simulink model "aero_gen"  (R2021b)
settings: Solver=ode45  StartTime=0.0  StopTime=inf  FixedStep=0.005  RelTol=1e-3
model workspace (MATLAB code in the model file + MAT data in the model file):
  | k = 110
values from neighbouring files (symbols this model uses):
  pitch_c = deg2rad(8)    [run_sim.m]    (also in run_sim_config.m = flight_config.aircraft_params.pitch_control_input; run_static_trim.m = deg2rad(-10))
  roll_c_1 = deg2rad(0)    [run_sim.m]    (also in run_sim_config.m = flight_config.aircraft_params.roll_control_input_1; run_static_trim.m = deg2rad(12.6))
  viz_on = 1    [run_sim.m]    (also in run_sim_config.m = flight_config.sys_params.viz_on; run_static_trim.m)
  yaw_moment_1 = 0.00    (= 0)    [run_sim.m]    (also in run_sim_config.m = flight_config.aircraft_params.yaw_moment_coeff_1; run_static_trim.m)
undefined symbols (not defined in the file or in its folder): state1
libraries: block_library x7, vrlib x1
settings Model: SnapshotBufferSize=1000  Creator=austm  LastModifiedBy=austm
settings SolverCC: ZeroCrossAlgorithm=Adaptive  AutoInsertRateTranBlk=on  InsertRTBMode=Never (minimum delay)  DecoupledContinuousIntegration=on  MinimalZcImpactIntegration=on
settings DataIOCC: ExternalInput=[0, u_trim']  InitialState=[x_trim']  LoadExternalInput=on  SaveFormat=Array  SaveOutput=off  ReturnWorkspaceOutputsName=tpc05cf441_1fa6_4e1e_817c_7c8b4b7bc3e9
settings OptimizationCC: EnhancedBackFolding=on  StrengthReduction=on  InitFltsAndDblsToZero=on  DifferentSizesBufferReuse=on
settings DebuggingCC: WriteAfterWriteMsg=DisableAll  AlgebraicLoopMsg=none  IgnoredZcDiagnostic=none  FcnCallInpInsideContextMsg=warning  UnconnectedInputMsg=none  UnconnectedOutputMsg=none  UnconnectedLineMsg=none  UniqueDataStoreMsg=error  RootOutportRequireBusObject=none  StrictBusMsg=ErrorOnBusTreatedAsVector  SFUnexpectedBacktrackingDiag=warning  SFNoUnconditionalDefaultTransitionDiag=warning  SFExecutionAtInitializationDiag=none  SFMachineParentedDataDiag=warning  ArithmeticOperatorsInVariantConditions=warning
settings ModelReferenceCC: PropagateSignalLabelsOutOfModel=off
settings SFSimCC: SimUseLocalCustomCode=off
settings RTWCC: RTWUseLocalCustomCode=off
settings CodeAppCC: StateflowObjectComments=on

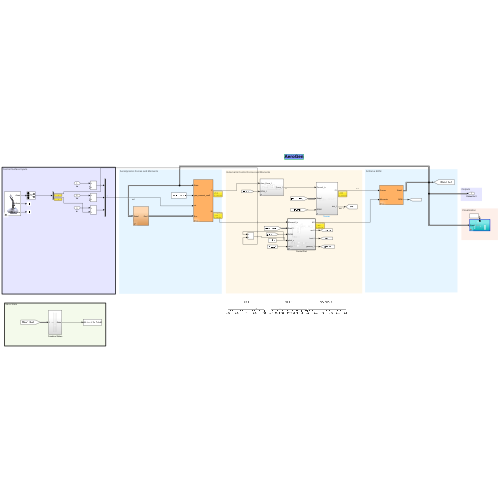
[thumbnail: Simulink's stored preview of the top-level diagram]
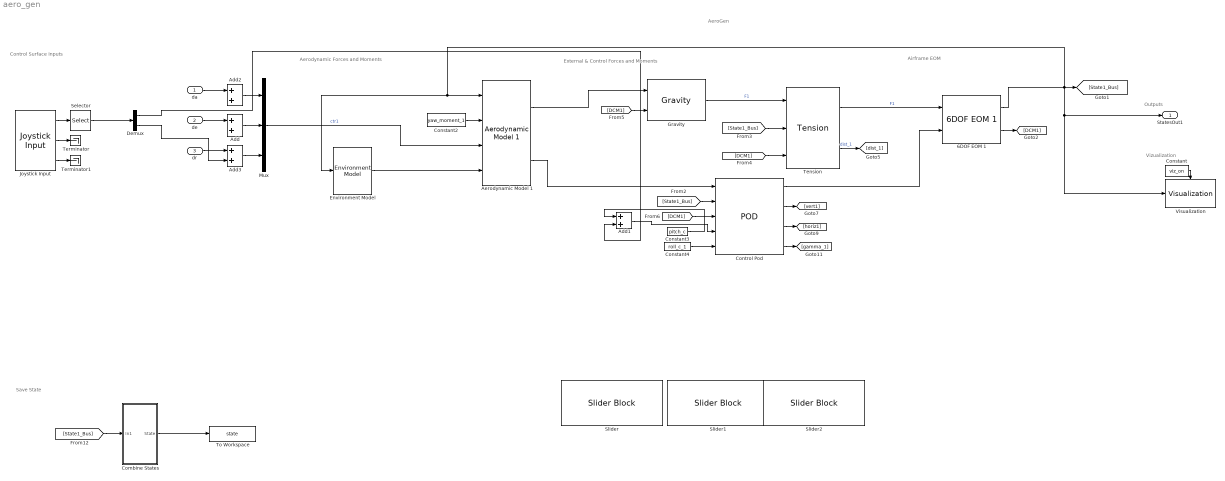
== system aero_gen ==
  note: Control Surface Inputs
  note: Save State
  note: AeroGen
  note: Airframe EOM
  note: Outputs
  note: Aerodynamic Forces and Moments
  note: Vizualization
  note: External & Control Forces and Moments
  da : Inport
  de : Inport  Port=2
  dr : Inport  Port=3
  6DOF EOM 1 : block_library/6DOF EOM 1  VariantControl=eom3DOF  XYZ=[state1.XN, state1.XE, state1.XD]  uvw=[state1.U, state1.V, state1.W]  rpy=[state1.Phi, state1.Theta, state1.Psi]  pqr=[state1.P, state1.Q, state1.R]  m=state1.Mass  I=state1.Inertia.Variables
  Add{,1..3} (4 alike) : Sum
  Aerodynamic Model 1 : block_library/Aerodynamic Model 1  VariantControl=aeroCONST  CG=state1.CenterOfGravity  CP=state1.CenterOfPressure
  Combine States : Subsystem
  Constant : Constant  Value=viz_on
  Constant2 : Constant  Value=yaw_moment_1
  Constant3 : Constant  Value=pitch_c
  Constant4 : Constant  Value=roll_c_1
  Control Pod : block_library/POD  SystemSampleTime=-1  VariantActivationTime=update diagram  Latency=0  AutoFrameSizeCalculation=off
  Demux : Demux  Outputs=2
  Environment Model : block_library/Environment Model  SystemSampleTime=-1  VariantControl=aeroCONST  VariantActivationTime=update diagram  Latency=0  AutoFrameSizeCalculation=off
  Gravity : block_library/Gravity  SystemSampleTime=-1  VariantActivationTime=update diagram  Latency=0  AutoFrameSizeCalculation=off
  Joystick Input : vrlib/Joystick Input  joyid=1  adjustports=on  forcefeed=off
  Mux : Mux  Inputs=3
  Selector : Selector  InputPortWidth=3  IndexOptions=Index vector (dialog)  Indices=[2, 1]  OutputSizes=1
  Slider : SliderBlock  ScaleMin=-.26  ScaleMax=.26
  Slider1 : SliderBlock  ScaleMin=-.17  ScaleMax=.5
  Slider2 : SliderBlock  ScaleMax=.1
  Tension : block_library/Tension  SystemSampleTime=-1  VariantActivationTime=update diagram  Latency=0  AutoFrameSizeCalculation=off
  Terminator : Terminator
  Terminator1 : Terminator
  To Workspace : ToWorkspace  VariableName=state  SaveFormat=Structure With Time  SampleTime=-1
  Visualization : block_library/Visualization  SystemSampleTime=-1  VariantActivationTime=update diagram  Latency=0  AutoFrameSizeCalculation=off
      link override VR Sink: SampleTime=0.02  RemoteView=off  FieldsWritten=aircraft_1.rotation.4.1.1.double#aircraft_1.translation.3.1.1.double  WorldFileName=aero_gen_virtual_environment.wrl  AutoView=off  VideoDimensions=[]  AllowVariableSize=off
  StatesOut1 : Outport  OutDataTypeStr=double  VectorParamsAs1DForOutWhenUnconnected=off
  wires:
  Control Pod/1 -> 6DOF EOM 1/2
  Tension/1 -> 6DOF EOM 1/1  "F1"
  Constant/1 -> Visualization/Enable
  Environment Model/1 -> Aerodynamic Model 1/4
  Gravity/1 -> Tension/1  "F1"
  Aerodynamic Model 1/1 -> Gravity/1
  Aerodynamic Model 1/2 -> Control Pod/1
  [State1_Bus] -> Control Pod/2
  [State1_Bus] -> Tension/2
  [DCM1] -> Tension/3
  [DCM1] -> Gravity/2
  [DCM1] -> Control Pod/3
  Constant2/1 -> Aerodynamic Model 1/2
  [State1_Bus] -> Combine States/1(In1)
  Mux/1 -> Aerodynamic Model 1/3  "ctr1"
  6DOF EOM 1/1 -> Environment Model/1, Aerodynamic Model 1/1, Visualization/1, StatesOut1/1, [State1_Bus]
  Tension/2 -> [dist_1]  "dist_1"
  Control Pod/2 -> [vert1]
  Control Pod/3 -> [horiz1]
  Constant3/1 -> Add1/1
  Constant4/1 -> Control Pod/5
  Combine States/1(State) -> To Workspace/1
  Add/1 -> Mux/2
  Add2/1 -> Mux/1
  Add3/1 -> Mux/3
  de/1 -> Add/1
  Control Pod/4 -> [gamma_1]
  dr/1 -> Add3/1
  6DOF EOM 1/2 -> [DCM1]
  da/1 -> Add2/1
  Joystick Input/1 -> Selector/1
  Joystick Input/2 -> Terminator/1
  Selector/1 -> Demux/1
  Joystick Input/3 -> Terminator1/1
  Demux/1 -> Add1/2
  Demux/2 -> Add3/2
  Add1/1 -> Control Pod/4

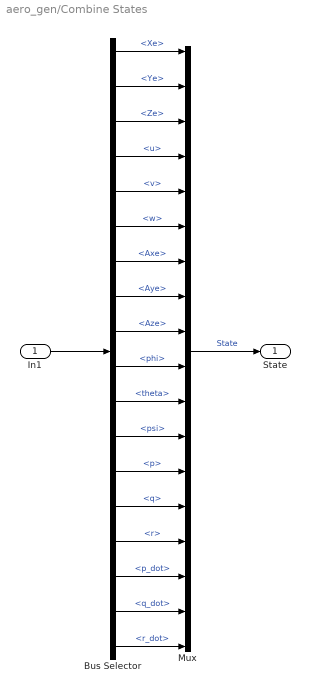
== system aero_gen/Combine States ==
  In1 : Inport
  Bus Selector : BusSelector  OutputSignals=Xe,Ye,Ze,u,v,w,Axe,Aye,Aze,phi,theta,psi,p,q,r,p_dot,q_dot,r_dot
  Mux : Mux  Inputs=18
  State : Outport
  wires:
  Bus Selector/10 -> Mux/10  "<phi>"
  Bus Selector/8 -> Mux/8  "<Aye>"
  Bus Selector/14 -> Mux/14  "<q>"
  Mux/1 -> State/1  "State"
  Bus Selector/1 -> Mux/1  "<Xe>"
  Bus Selector/11 -> Mux/11  "<theta>"
  Bus Selector/7 -> Mux/7  "<Axe>"
  Bus Selector/12 -> Mux/12  "<psi>"
  Bus Selector/4 -> Mux/4  "<u>"
  Bus Selector/9 -> Mux/9  "<Aze>"
  Bus Selector/17 -> Mux/17  "<q_dot>"
  Bus Selector/5 -> Mux/5  "<v>"
  Bus Selector/15 -> Mux/15  "<r>"
  Bus Selector/3 -> Mux/3  "<Ze>"
  Bus Selector/2 -> Mux/2  "<Ye>"
  Bus Selector/13 -> Mux/13  "<p>"
  Bus Selector/6 -> Mux/6  "<w>"
  Bus Selector/16 -> Mux/16  "<p_dot>"
  Bus Selector/18 -> Mux/18  "<r_dot>"
  In1/1 -> Bus Selector/1
